simulink model "inv_objfunc"  (R2023a)
settings: Solver=FixedStepAuto  StartTime=0.0  StopTime=10.0  RelTol=1e-3
values from neighbouring files (symbols this model uses):
  globalBest = particles(i, :)    [pso_code.m]
libraries: spsIGBTDiodeLib x12, simulink x6, spsFourierLib x4, spsDCVoltageSourceLib x3, spsSeriesRLCBranchLib x1, spsVoltageMeasurementLib x1, spspowerguiLib x1
settings Model: Creator=jain  LastModifiedBy=banof
settings DebuggingCC: UnconnectedInputMsg=warning  UnconnectedOutputMsg=warning  UnconnectedLineMsg=warning
settings ModelReferenceCC: EnableRefExpFcnMdlSchedulingChecks=on
settings RTWCC: DLArmComputeVersion=19.05

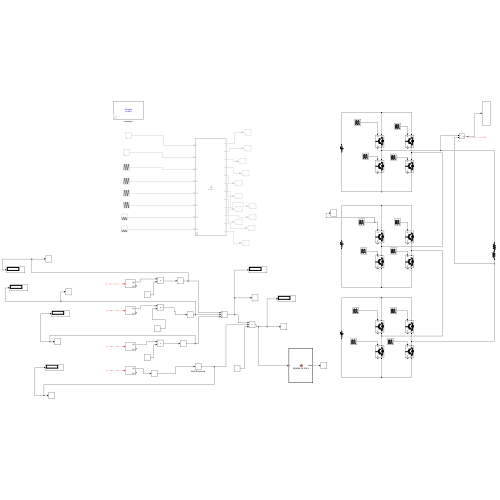
[thumbnail: Simulink's stored preview of the top-level diagram]
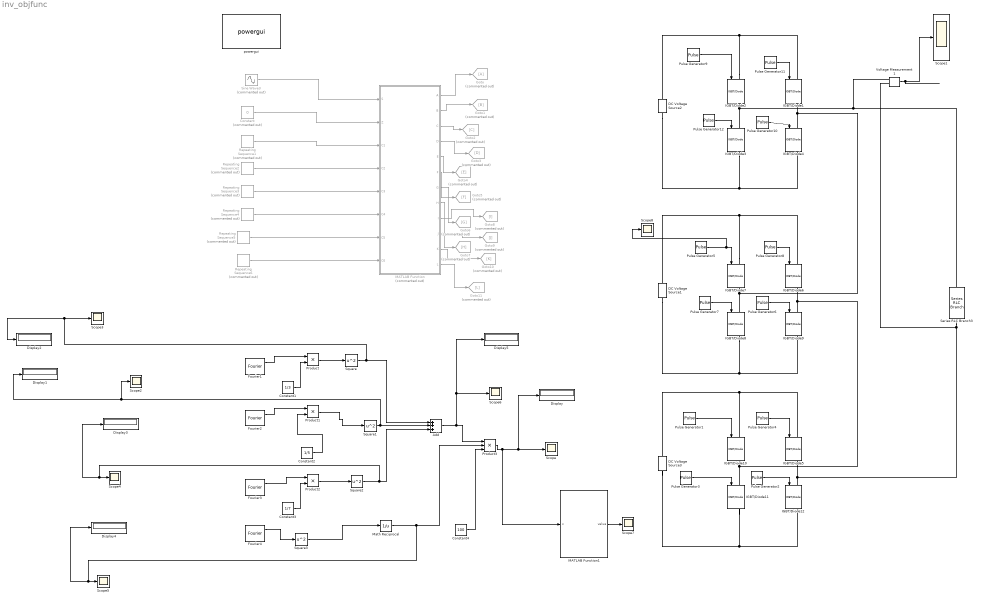
== system inv_objfunc ==
  Add : Sum  Inputs=+++
  Constant : Constant  Commented=on  Value=0
  Constant1 : Constant  Value=1/3
  Constant2 : Constant  Value=1/5
  Constant3 : Constant  Value=1/7
  Constant4 : Constant  Value=100
  DC Voltage Source1 : spsDCVoltageSourceLib/DC Voltage Source  Amplitude=100  Measurements=None
  DC Voltage Source2 : spsDCVoltageSourceLib/DC Voltage Source  Amplitude=100  Measurements=None
  DC Voltage Source3 : spsDCVoltageSourceLib/DC Voltage Source  Amplitude=100  Measurements=None
  Display{,1..5} (6 alike) : Display
  Fourier1 : spsFourierLib/Fourier  Freq=50  n=3  InInit=[0, 0]  Ts=0
  Fourier2 : spsFourierLib/Fourier  Freq=50  n=5  InInit=[0, 0]  Ts=0
  Fourier3 : spsFourierLib/Fourier  Freq=50  n=7  InInit=[0, 0]  Ts=0
  Fourier4 : spsFourierLib/Fourier  Freq=50  n=1  InInit=[0, 0]  Ts=0
  Goto : Goto  Commented=on
  Goto1 : Goto  Commented=on  GotoTag=B
  Goto10 : Goto  Commented=on  GotoTag=K
  Goto11 : Goto  Commented=on  GotoTag=L
  Goto2 : Goto  Commented=on  GotoTag=C
  Goto3 : Goto  Commented=on  GotoTag=D
  Goto4 : Goto  Commented=on  GotoTag=E
  Goto5 : Goto  Commented=on  GotoTag=F
  Goto6 : Goto  Commented=on  GotoTag=G
  Goto7 : Goto  Commented=on  GotoTag=H
  Goto8 : Goto  Commented=on  GotoTag=I
  Goto9 : Goto  Commented=on  GotoTag=J
  IGBT/Diode{1..12} (12 alike) : spsIGBTDiodeLib/IGBT//Diode  Ron=1e-3  Rs=1e5  Cs=inf  Measurements=on
  MATLAB Function : MATLAB Function  Commented=on  TreatAsAtomicUnit=on
  MATLAB Function1 : MATLAB Function  TreatAsAtomicUnit=on
  Math Reciprocal : Math  Operator=reciprocal  SignedPower=on
  Product : Product
  Product1 : Product
  Product2 : Product
  Product3 : Product  Inputs=3
  Pulse Generator1 : DiscretePulseGenerator  PulseType=Time based  Period=.02  PulseWidth=(180-2*globalBest(1))*100/360  PhaseDelay=globalBest(1)*0.02/360
  Pulse Generator10 : DiscretePulseGenerator  PulseType=Time based  Period=.02  PulseWidth=(180-2*globalBest(3))*100/360  PhaseDelay=globalBest(3)*0.02/360
  Pulse Generator11 : DiscretePulseGenerator  PulseType=Time based  Period=.02  PulseWidth=(180-2*globalBest(3))*100/360  PhaseDelay=(180+globalBest(3))*0.02/360
  Pulse Generator12 : DiscretePulseGenerator  PulseType=Time based  Period=.02  PulseWidth=(180-2*globalBest(3))*100/360  PhaseDelay=(180+globalBest(3))*0.02/360
  Pulse Generator2 : DiscretePulseGenerator  PulseType=Time based  Period=.02  PulseWidth=(180-2*globalBest(1))*100/360  PhaseDelay=globalBest(1)*0.02/360
  Pulse Generator3 : DiscretePulseGenerator  PulseType=Time based  Period=.02  PulseWidth=(180-2*globalBest(1))*100/360  PhaseDelay=(180+globalBest(1))*0.02/360
  Pulse Generator4 : DiscretePulseGenerator  PulseType=Time based  Period=.02  PulseWidth=(180-2*globalBest(1))*100/360  PhaseDelay=(180+globalBest(1))*0.02/360
  Pulse Generator5 : DiscretePulseGenerator  PulseType=Time based  Period=.02  PulseWidth=(180-2*globalBest(2))*100/360  PhaseDelay=globalBest(2)*0.02/360
  Pulse Generator6 : DiscretePulseGenerator  PulseType=Time based  Period=.02  PulseWidth=(180-2*globalBest(2))*100/360  PhaseDelay=globalBest(2)*0.02/360
  Pulse Generator7 : DiscretePulseGenerator  PulseType=Time based  Period=.02  PulseWidth=(180-2*globalBest(2))*100/360  PhaseDelay=(180+globalBest(1))*0.02/360
  Pulse Generator8 : DiscretePulseGenerator  PulseType=Time based  Period=.02  PulseWidth=(180-2*globalBest(2))*100/360  PhaseDelay=(180+globalBest(2))*0.02/360
  Pulse Generator9 : DiscretePulseGenerator  PulseType=Time based  Period=.02  PulseWidth=(180-2*globalBest(3))*100/360  PhaseDelay=globalBest(3)*0.02/360
  Repeating Sequence1 : simulink/Sources/Repeating Sequence  Commented=on  rep_seq_t=[0 0.5/1000 1/1000]  rep_seq_y=[0 0.3334 0]
  Repeating Sequence2 : simulink/Sources/Repeating Sequence  Commented=on  rep_seq_t=[0 0.5/1000 1/1000]  rep_seq_y=[0.3334 0.6667 0.3334]
  Repeating Sequence3 : simulink/Sources/Repeating Sequence  Commented=on  rep_seq_t=[0 0.5/1000 1/1000]  rep_seq_y=[0.6667 1.0000 0.6667]
  Repeating Sequence4 : simulink/Sources/Repeating Sequence  Commented=on  rep_seq_t=[0 0.5/1000 1/1000]  rep_seq_y=[0 -0.3334 0]
  Repeating Sequence5 : simulink/Sources/Repeating Sequence  Commented=on  rep_seq_t=[0 0.5/1000 1/1000]  rep_seq_y=[-0.3334 -0.6667 -0.3334]
  Repeating Sequence6 : simulink/Sources/Repeating Sequence  Commented=on  rep_seq_t=[0 0.5/1000 1/1000]  rep_seq_y=[-0.6667 -1 -0.6667]
  Scope{,1..8} (9 alike) : Scope
  Series RLC Branch3 : spsSeriesRLCBranchLib/Series RLC Branch  LConnTagsString=__new0  RConnTagsString=__new0  BranchType=RL  Resistance=100  Inductance=100e-3  SetiL0=off  InitialCurrent=0  Capacitance=1e-6  Setx0=off  InitialVoltage=0  Measurements=None
  Sine Wave3 : Sin  Commented=on  Frequency=2*pi*50
  Square{,1..3} (4 alike) : Math  Operator=square
  Voltage Measurement1 : spsVoltageMeasurementLib/Voltage Measurement  PhasorSimulation=off  OutputType=Complex  PSBequivalent=0
  powergui : spspowerguiLib/powergui  Priority=1  SimulationMode=Discrete  SampleTime=1e-6  frequency=60  Iterations=50  frequencyindice=0  Pbase=100e6  ErrMax=1e-4  UnitsV=kV  UnitsW=MW  buscounter=0  FunctionMessages=off  echomessages=off  EnableUseOfTLC=off  CurrentSourceSwitches=off  DisableSnubberDevices=off  DisableRonSwitches=off  DisableVfSwitches=off  DisplayEquations=off  AutomaticDiscreteSolvers=off  SolverType=Tustin/Backward Euler (TBE)  Interpol=off  ExternalGateDelay=off  methode=off  Ts=100  x0status=blocks  SPID=on  SwTol=0  HookPort=off  NonlinearTolerance=1e-4  nMaxIteration=100  ContinueOnMaxIteration=off  RestoreLinks=warning  ResistiveCurrentMeasurement=off  Frange=[0:2:500]  Ylog=off  Xlog=on  ShowGrid=off  save=off  variable=ZData  structure=0  ZoomFFT=off  StartTime=0.0  cycles=1  DisplayStyle=1  fundamental=60  FreqAxis=off  MaxFrequency=1000  frequencyindicesteady=1  RmsSteady=1  display=off
  wires:
  Pulse Generator8/1 -> IGBT/Diode6/1
  Pulse Generator5/1 -> Scope8/1, IGBT/Diode7/1
  Pulse Generator7/1 -> IGBT/Diode8/1
  Pulse Generator6/1 -> IGBT/Diode9/1
  Pulse Generator11/1 -> IGBT/Diode1/1
  Pulse Generator12/1 -> IGBT/Diode3/1
  Pulse Generator9/1 -> IGBT/Diode2/1
  Pulse Generator10/1 -> IGBT/Diode4/1
  MATLAB Function/1(A) -> Goto/1
  MATLAB Function/2(B) -> Goto1/1
  MATLAB Function/3(C) -> Goto2/1
  MATLAB Function/4(D) -> Goto3/1
  MATLAB Function/5(E) -> Goto4/1
  MATLAB Function/6(F) -> Goto5/1
  MATLAB Function/7(G) -> Goto6/1
  MATLAB Function/8(H) -> Goto7/1
  Voltage Measurement1/1 -> Scope1/1
  Pulse Generator3/1 -> IGBT/Diode11/1
  Pulse Generator2/1 -> IGBT/Diode12/1
  Pulse Generator1/1 -> IGBT/Diode10/1
  Pulse Generator4/1 -> IGBT/Diode5/1
  MATLAB Function/9(I) -> Goto8/1
  MATLAB Function/11(K) -> Goto10/1
  MATLAB Function/12(L) -> Goto11/1
  Repeating Sequence4/1 -> MATLAB Function/6(C4)
  Repeating Sequence5/1 -> MATLAB Function/7(C5)
  Repeating Sequence6/1 -> MATLAB Function/8(C6)
  MATLAB Function/10(J) -> Goto9/1
  Repeating Sequence3/1 -> MATLAB Function/5(C3)
  Repeating Sequence2/1 -> MATLAB Function/4(C2)
  Repeating Sequence1/1 -> MATLAB Function/3(C1)
  Sine Wave3/1 -> MATLAB Function/1(S)
  Constant/1 -> MATLAB Function/2(Z)
  Fourier1/1 -> Product/1
  Constant1/1 -> Product/2
  Product/1 -> Square/1
  Fourier2/1 -> Product1/1
  Constant2/1 -> Product1/2
  Product2/1 -> Square2/1
  Fourier3/1 -> Product2/1
  Constant3/1 -> Product2/2
  Fourier4/1 -> Square3/1
  Square1/1 -> Display1/1, Scope2/1, Add/2
  Square3/1 -> Math Reciprocal/1
  Constant4/1 -> Product3/3
  Product3/1 -> MATLAB Function1/1(x), Scope/1, Display/1
  ? -> Fourier1/1
  ? -> Fourier2/1
  ? -> Fourier3/1
  ? -> Fourier4/1
  Product1/1 -> Square1/1
  Square/1 -> Add/1, Scope3/1, Display2/1
  Square2/1 -> Display3/1, Scope4/1, Add/3
  Math Reciprocal/1 -> Display4/1, Scope5/1, Product3/2
  Add/1 -> Scope6/1, Display5/1, Product3/1
  MATLAB Function1/1(value) -> Scope7/1
  connections:
  IGBT/Diode7/LConn1 -- IGBT/Diode6/LConn1 -- DC Voltage Source1/RConn1
  DC Voltage Source1/LConn1 -- IGBT/Diode9/RConn1 -- IGBT/Diode8/RConn1
  IGBT/Diode2/LConn1 -- IGBT/Diode1/LConn1 -- DC Voltage Source2/RConn1
  IGBT/Diode2/RConn1 -- Voltage Measurement1/LConn1 -- Series RLC Branch3/LConn1 -- IGBT/Diode3/LConn1
  DC Voltage Source2/LConn1 -- IGBT/Diode4/RConn1 -- IGBT/Diode3/RConn1
  IGBT/Diode11/RConn1 -- IGBT/Diode12/RConn1 -- DC Voltage Source3/LConn1
  DC Voltage Source3/RConn1 -- IGBT/Diode5/LConn1 -- IGBT/Diode10/LConn1
  IGBT/Diode5/RConn1 -- Voltage Measurement1/LConn2 -- Series RLC Branch3/RConn1 -- IGBT/Diode12/LConn1
  IGBT/Diode4/LConn1 -- IGBT/Diode8/LConn1 -- IGBT/Diode7/RConn1 -- IGBT/Diode1/RConn1
  IGBT/Diode9/LConn1 -- IGBT/Diode10/RConn1 -- IGBT/Diode11/LConn1 -- IGBT/Diode6/RConn1

== matlab function inv_objfunc/MATLAB Function1 ==
  data: x input; value output
function value = objectiveFunction(x)
    value = x;
end

== matlab function inv_objfunc/MATLAB Function ==
  data: S input; A output; B output; C output; D output; E output; F output; G output; H output; I output; J output; K output; L output; Z input; C1 input; C2 input; C3 input; C4 input; C5 input; C6 input
function [A,B,C,D,E,F,G,H,I,J,K,L]= myfcn(S,Z,C1,C2,C3,C4,C5,C6)
    a=0;b=0;c=0;d=0;e=0;f=0;g=0;h=0;i=0;j=0;k=0;l=0;
if S>Z&&S>C1&&S<C2&&S<C3%1/3Vdc
    a=1;
    b=0;
    c=0;
    d=1;
    e=1;
    f=0;
    g=1;
    h=0;
    i=1;
    j=0;
    k=1;
    l=0;
elseif S>Z&&S>C1&&S>C2&&S<C3%2/3Vdc
    a=1;
    b=0;
    c=1;
    d=0;
    e=1;
    f=0;
    g=0;
    h=1;
    i=1;
    j=0;
    k=0;
    l=1;
elseif S>Z&&S>C1&&S>C2&&S>C3%VDC
    a=1;
    b=0;
    c=0;
    d=1;
    e=1;
    f=0;
    g=0;
    h=1;
    i=1;
    j=0;
    k=0;
    l=1;
  elseif S>Z&&S<C1&&S<C2&&S<C3%0Vdc
    a=1;
    b=0;
    c=1;
    d=0;
    e=1;
    f=0;
    g=1;
    h=0;    
    i=1;
    j=0;
    k=1;
    l=0;
elseif S<Z&&S>C4&&S>C5&&S>C6%0Vdc
    a=1;
    b=0;
    c=1;
    d=0;
    e=1;
    f=0;
    g=1;
    h=0;    
    i=1;
    j=0;
    k=1;
    l=0;
    elseif S<Z&&S<C4&&S>C5&&S>C6%-1/3Vdc
    a=0;
    b=1;
    c=1;
    d=0;
    e=1;
    f=0;
    g=1;
    h=0;    
    i=1;
    j=0;
    k=1;
    l=0;
    elseif S<Z&&S<C4&&S<C5&&S>C6%-2/3Vdc
    a=0;
    b=1;
    c=1;
    d=0;
    e=0;
    f=1;
    g=1;
    h=0;    
    i=1;
    j=0;
    k=1;
    l=0;
    elseif S<Z&&S<C4&&S<C5&&S<C6%-Vdc
    a=0;
    b=1;
    c=1;
    d=0;
    e=0;
    f=1;
    g=1;
    h=0;    
    i=0;
    j=1;
    k=1;
    l=0;
end
A=a;
B=b;
C=c;
D=d;
E=e;
F=f;
G=g;
H=h;
I=i;
J=j;
K=k;
L=l;
